simulink subsystem "Humid_Control"  (R2024b)
settings: Solver=VariableStepAuto  StartTime=0.0  StopTime=10.0  RelTol=1e-3
libraries: slident x1
settings Model: DataDictionary=Humidifier_Interface.sldd  EnableAccessToBaseWorkspace=off  Creator=ppatel  LastModifiedBy=ppatel

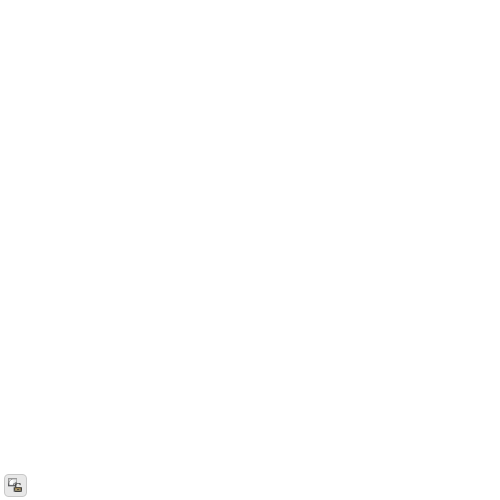
[thumbnail: Simulink's stored preview of the top-level diagram]
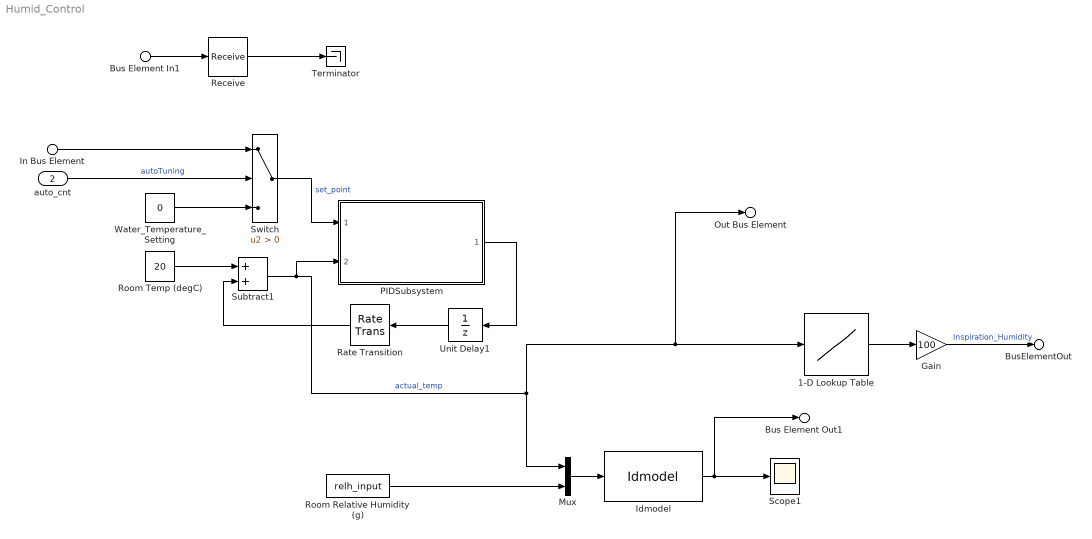
== system Humid_Control ==
  Bus Element In1 : Inport  OutputPortMessageModes=m  PortName=HumidityAdj
  auto_cnt : Inport  Port=2
  In Bus Element : Inport  Port=3  PortName=humid  Element=Humidity
  1-D Lookup Table : Lookup_n-D  NumberOfTableDimensions=1  BreakpointsForDimension1=[20 25 30 35 40 45]  Table=[0.25 0.3 0.375 0.475 0.6 0.7]  InternalRulePriority=Speed  RndMeth=Simplest
  Gain : Gain  Gain=100
  Idmodel : slident/Models/Idmodel  sys=mp  IC=0  noi=on  seed=[]
  Mux : Mux  Inputs=2
  PIDSubsystem : Subsystem  ClipboardFcn=|  SystemSampleTime=0.05  ReferencedSubsystem=PIDSubsystem
      | Ts = 0.05;
      | Kp = 0.1;
      | Ki = 0.5;
      settings: PermitHierarchicalResolution=None
  Rate Transition : RateTransition
  Receive : Receive  InputPortMessageModes=m  UseInternalQueue=off  QueueOverwriting=on  QueueLength=1  QueueType=LIFO
  Room Relative Humidity (g) : FromWorkspace  VariableName=relh_input  OutDataTypeStr=double
  Room Temp (degC) : Constant  Value=20
  Scope1 : Scope
  Subtract1 : Sum
  Switch : Switch  Criteria=u2 > Threshold  SaturateOnIntegerOverflow=off  InputSameDT=off
  Terminator : Terminator
  Unit Delay1 : UnitDelay  SampleTime=0.05  HasFrameUpgradeWarning=on
  Water_Temperature_Setting : Constant  Value=0
  Bus Element Out1 : Outport  PortName=HumidH  Element=Humidifier_H
  BusElementOut : Outport  PortName=HumidH  Element=Insp_Humidity
  Out Bus Element : Outport  Port=2  PortName=Thermistor  Element=Water_T
  wires:
  In Bus Element/1 -> Switch/1
  Subtract1/1 -> PIDSubsystem/2, Mux/1, Out Bus Element/1, 1-D Lookup Table/1  "actual_temp"
  Mux/1 -> Idmodel/1
  Idmodel/1 -> Scope1/1, Bus Element Out1/1
  Unit Delay1/1 -> Rate Transition/1
  Switch/1 -> PIDSubsystem/1  "set_point"
  Water_Temperature_Setting/1 -> Switch/3
  1-D Lookup Table/1 -> Gain/1
  Room Relative Humidity (g)/1 -> Mux/2
  Gain/1 -> BusElementOut/1  "Inspiration_Humidity"
  auto_cnt/1 -> Switch/2  "autoTuning"
  Room Temp (degC)/1 -> Subtract1/1
  PIDSubsystem/1 -> Unit Delay1/1
  Rate Transition/1 -> Subtract1/2
  Bus Element In1/1 -> Receive/1
  Receive/1 -> Terminator/1
